simulink model "sim_arm_sfbk_R2013a"  (R2013a)
settings: Solver=ode4  SolverMode=SingleTasking  StartTime=0.0  StopTime=1  FixedStep=0.001  RelTol=1e-3
values from neighbouring files (symbols this model uses):
  A = [    0       1 ... (first row only)    [arm_acker.m]    (also in arm_acker_R2013a.m; arm_acker_R2015a.m; arm_acker_R2018a.m; arm_acker_custom.m)
  B = [ 0 ... (first row only)    [arm_acker.m]    (also in arm_acker_R2013a.m; arm_acker_R2015a.m; arm_acker_R2018a.m; arm_acker_custom.m)
  K = - acker(A,B,p)    [arm_acker.m]    (also in arm_acker_R2013a.m; arm_acker_R2015a.m; arm_acker_R2018a.m; arm_acker_custom.m)
  x0 = [ 1  0 ]'    [arm_acker.m]    (also in arm_acker_R2013a.m; arm_acker_R2015a.m; arm_acker_R2018a.m; arm_acker_custom.m)
settings Model: CovMetricSettings=dwe  CovHtmlReporting=off  covSaveCumulativeToWorkspaceVar=off  CovSaveSingleToWorkspaceVar=off  CovExternalEMLEnable=on  Creator=kawata  LastModifiedBy=kawata
settings DataIOCC: LimitDataPoints=off  SaveFormat=StructureWithTime
settings DebuggingCC: UnderspecifiedInitializationDetection=Simplified  MergeDetectMultiDrivingBlocksExec=error  SolverPrmCheckMsg=none  FrameProcessingCompatibilityMsg=error  StateNameClashWarn=none  SFUnexpectedBacktrackingDiag=error  SFNoUnconditionalDefaultTransitionDiag=error
settings HardwareCC: ProdBitPerPointer=64  ProdLargestAtomicFloat=Float  ProdIntDivRoundTo=Zero  ProdEndianess=LittleEndian  ProdHWDeviceType=Specified
settings ModelReferenceCC: PropagateSignalLabelsOutOfModel=on
settings GRTTargetCC: CodeReplacementLibrary=C99 (ISO)  GeneratePreprocessorConditionals=Use local settings

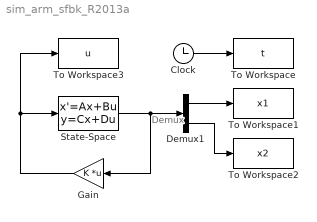
== system sim_arm_sfbk_R2013a ==
  note: Demux
  Clock : Clock
  Demux1 : Demux  Outputs=2
  Gain : Gain  Gain=K  Multiplication=Matrix(K*u)
  State-Space : StateSpace  A=A  B=B  C=eye(2)  D=zeros(2,1)  X0=x0
  To Workspace : ToWorkspace  VariableName=t  SampleTime=-1
  To Workspace1 : ToWorkspace  VariableName=x1  SampleTime=-1
  To Workspace2 : ToWorkspace  VariableName=x2  SampleTime=-1
  To Workspace3 : ToWorkspace  VariableName=u  SampleTime=-1
  wires:
  State-Space/1 -> Gain/1, Demux1/1
  Gain/1 -> To Workspace3/1, State-Space/1
  Clock/1 -> To Workspace/1
  Demux1/1 -> To Workspace1/1
  Demux1/2 -> To Workspace2/1
